simulink model "a"  (R2013a)
settings: Solver=VariableStepDiscrete  StartTime=0.0  StopTime=9  RelTol=1e-3
undefined symbols (not defined in the file): Ts
libraries: powerlib x2, electricdrivelib x1, simulink x1
settings Model: Creator=Guilherme  LastModifiedBy=Guilherme

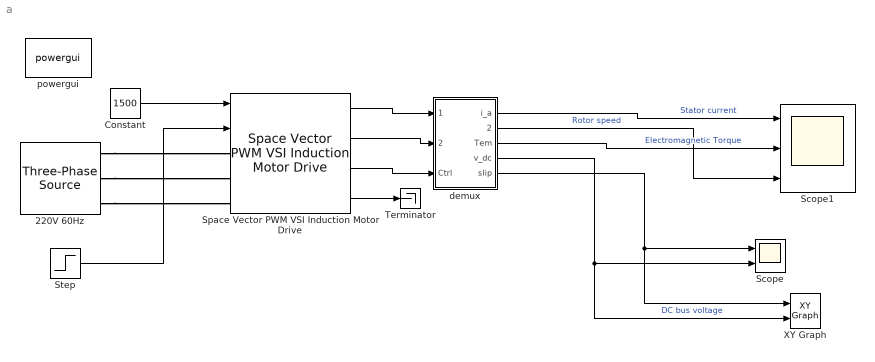
== system a ==
  220V 60Hz : powerlib/Electrical Sources/Three-Phase Source  Voltage=220  PhaseAngle=0  Frequency=60  InternalConnection=Yg  SpecifyImpedance=off  Resistance=0.02  Inductance=0.05e-3  ShortCircuitLevel=100e6  BaseVoltage=25e3  XRratio=7  BusType=swing  Pref=0  Qref=0  Qmin=-inf  Qmax=inf
  Constant : Constant  Value=1500
  Scope : Scope  NumInputPorts=2
      settings: YMin=0.989~302.5  YMax=1.002~322.5  Decimation=100
  Scope1 : Scope  NumInputPorts=3
      settings: TimeRange=9  YMin=-12.5~1~950  YMax=12.5~7.5~1600  Decimation=100
  Space Vector PWM VSI Induction Motor Drive : electricdrivelib/AC drives/Space Vector PWM VSI Induction Motor Drive  showMaskWarnings=on  AverageValue=on  MechanicalLoad=Torque Tm  driveType=AC2
  Step : Step  Time=6  Before=1  After=5.5  SampleTime=0
  Terminator : Terminator
  XY Graph : simulink/Sinks/XY Graph  xmin=0  xmax=1  ymin=300  ymax=350  st=-1
  demux : Subsystem
  powergui : powerlib/powergui  Priority=1  SimulationMode=Discrete  SolverType=Tustin  SampleTime=Ts*10  frequency=60  SPID=off  DisableSnubberDevices=off  DisableRonSwitches=off  DisableVfSwitches=off  SwTol=0  Interpol=off  DisplayEquations=off  frequencyindice=60  Pbase=100e6  ErrMax=1e-4  Iterations=50  UnitsV=kV  UnitsW=MW  FunctionMessages=off  echomessages=off  HookPort=off  EnableUseOfTLC=off  x0status=blocks  RestoreLinks=warning  ResistiveCurrentMeasurement=off  Frange=[0:2:500]  Ylog=off  Xlog=on  ShowGrid=off  save=off  variable=ZData  ZoomFFT=off  StartTime=0.0  cycles=1  DisplayStyle=1  fundamental=60  FreqAxis=off  MaxFrequency=1000  frequencyindicesteady=1  RmsSteady=1  display=off  Ts=0  methode=off
  wires:
  Step/1 -> Space Vector PWM VSI Induction Motor Drive/2
  Constant/1 -> Space Vector PWM VSI Induction Motor Drive/1
  demux/1(i_a) -> Scope1/1  "Stator current"
  demux/2(speed) -> Scope1/3  "Rotor speed"
  demux/3(Tem) -> Scope1/2  "Electromagnetic Torque"
  demux/4(v_dc) -> Scope/2, XY Graph/2  "DC bus voltage"
  Space Vector PWM VSI Induction Motor Drive/1 -> demux/1(Motor)
  Space Vector PWM VSI Induction Motor Drive/2 -> demux/2(Conv.)
  Space Vector PWM VSI Induction Motor Drive/3 -> demux/3(Ctrl)
  demux/5(slip) -> Scope/1, XY Graph/1
  Space Vector PWM VSI Induction Motor Drive/4 -> Terminator/1
  connections:
  220V 60Hz/RConn2 -- Space Vector PWM VSI Induction Motor Drive/LConn2
  220V 60Hz/RConn3 -- Space Vector PWM VSI Induction Motor Drive/LConn3
  220V 60Hz/RConn1 -- Space Vector PWM VSI Induction Motor Drive/LConn1

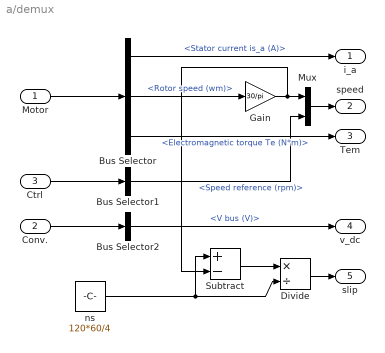
== system a/demux ==
  Motor : Inport
  Conv. : Inport  Port=2
  Ctrl : Inport  Port=3
  Bus Selector : BusSelector  OutputSignals=Stator measurements.Stator current is_a (A),Mechanical.Rotor speed (wm),Mechanical.Electromagnetic torque Te (N*m)
  Bus Selector1 : BusSelector  OutputSignals=Speed reference (rpm)
  Bus Selector2 : BusSelector  OutputSignals=V bus (V)
  Divide : Product  Inputs=*/
  Gain : Gain  Gain=30/pi  SaturateOnIntegerOverflow=on  OutDataTypeStr=Inherit: Same as input  ParamDataTypeStr=Inherit: Same as input
  Mux : Mux  Inputs=2
  Subtract : Sum  Inputs=+-
  ns : Constant  Value=120*60/4
  i_a : Outport
  speed : Outport  Port=2
  Tem : Outport  Port=3
  v_dc : Outport  Port=4
  slip : Outport  Port=5
  wires:
  Ctrl/1 -> Bus Selector1/1
  Gain/1 -> Subtract/2, Mux/1
  Mux/1 -> speed/1
  Motor/1 -> Bus Selector/1
  Bus Selector/1 -> i_a/1  "<Stator current is_a (A)>"
  Bus Selector/2 -> Gain/1  "<Rotor speed (wm)>"
  Bus Selector/3 -> Tem/1  "<Electromagnetic torque Te (N*m)>"
  Bus Selector1/1 -> Mux/2  "<Speed reference (rpm)>"
  Conv./1 -> Bus Selector2/1
  Bus Selector2/1 -> v_dc/1  "<V bus (V)>"
  ns/1 -> Divide/2, Subtract/1
  Subtract/1 -> Divide/1
  Divide/1 -> slip/1
